simulink model "Bloques"  (R2019a)
settings: Solver=VariableStepAuto  StartTime=0.0  StopTime=4000  RelTol=1e-3
values from neighbouring files (symbols this model uses):
  A = [0 1 0;0 0 1;-6 7 0]    [ParaCalcularLaP2.m]    (also in ParametrosBloques.m = [-(h21*A21+ha1*Aa1)/(m1*c1) (h21*A21)/(m1*c1) 0;(h12*A12)/(m)
  B = [Q/(m1*c1);0;0]    [ParametrosBloques.m]
  C = [1 0 0;0 1 0;0 0 1]    [ParametrosBloques.m]
  D = [0;0;0]    [ParametrosBloques.m]
  t0 = [298;295;293]    [ParametrosBloques.m]
  Xa = [293*(ha1*Aa1)/(m1*c1);0;0]    [ParametrosBloques.m]
settings Model: Creator=joaqu  LastModifiedBy=joaqu

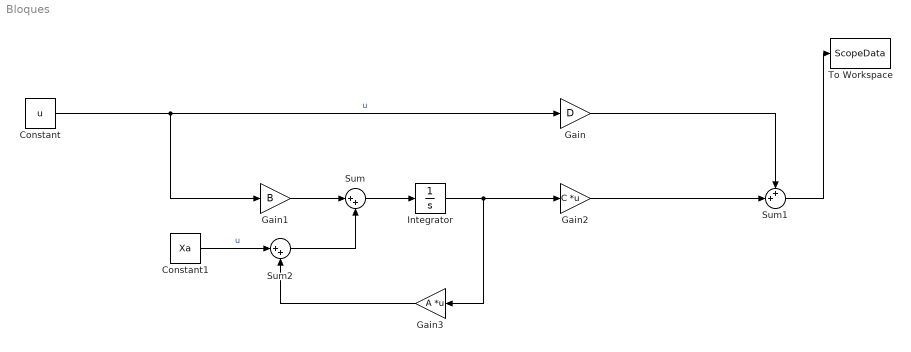
== system Bloques ==
  Constant : Constant  Value=u
  Constant1 : Constant  Value=Xa
  Gain : Gain  Gain=D
  Gain1 : Gain  Gain=B
  Gain2 : Gain  Gain=C  Multiplication=Matrix(K*u)
  Gain3 : Gain  Gain=A  Multiplication=Matrix(K*u)
  Integrator : Integrator  InitialCondition=t0
  Sum : Sum  Inputs=|++
  Sum1 : Sum  Inputs=++|
  Sum2 : Sum  Inputs=|++
  To Workspace : ToWorkspace  VariableName=ScopeData  SaveFormat=Structure With Time  SampleTime=-1
  wires:
  Constant/1 -> Gain/1, Gain1/1  "u"
  Integrator/1 -> Gain3/1, Gain2/1
  Sum/1 -> Integrator/1
  Sum1/1 -> To Workspace/1
  Gain2/1 -> Sum1/2
  Gain/1 -> Sum1/1
  Gain3/1 -> Sum2/2
  Gain1/1 -> Sum/1
  Sum2/1 -> Sum/2
  Constant1/1 -> Sum2/1  "u"
